simulink model "Male_female"  (R2017a)
settings: Solver=VariableStepAuto  StartTime=0.0  StopTime=10.0  RelTol=1e-3
libraries: dspvision x1
settings Model: Creator=harsh  LastModifiedBy=harsh

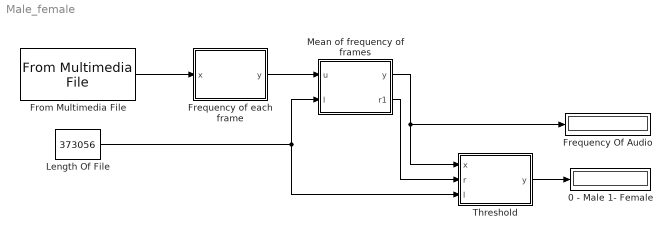
== system Male_female ==
  0 - Male 1- Female : Display
  Frequency Of Audio : Display
  Frequency of each frame : MATLAB Function  TreatAsAtomicUnit=on
  From Multimedia File : dspvision/From Multimedia File  inputFilename=E:\LNMIIT Study\Sem 5\Labs\DSP\Website\DSP Lab\Project (Male - Female Voice Recognition)\Project\samples\m2.wav  loop=on  numPlays=inf  outputStreams=Audio only  videoDataType=single  audioDataType=single  inheritSampleTime=on  userDefinedSampleTime=1/30  noAudioOutput=off  isIntensityVideo=off  fourcc=RGB  colorVideoFormat=Separate color signals  outputEOF=off  dataOrg=Column-major  audioFrameSize=3500  computeAudioFrameSize=off  outSamplingMode=Sample based
      settings: SourceProductBaseCode=VP
  "Length Of File " : Constant  Value=373056
  Mean of frequency of frames : MATLAB Function  TreatAsAtomicUnit=on
  Threshold : MATLAB Function  TreatAsAtomicUnit=on
  wires:
  From Multimedia File/1 -> Frequency of each frame/1(x)
  Frequency of each frame/1(y) -> Mean of frequency of frames/1(u)
  Mean of frequency of frames/1(y) -> Frequency Of Audio/1, Threshold/1(x)
  "Length Of File "/1 -> Threshold/3(l), Mean of frequency of frames/2(l)
  Threshold/1(y) -> 0 - Male 1- Female/1
  Mean of frequency of frames/2(r1) -> Threshold/2(r)

== matlab function Male_female/Threshold ==
  data: x input; r input; y output; l input
function y = fcn(x,r,l)
y=5;
if r>l/3500
    if x>160
        y=1;
    else
        y=0;
    end
end
end

== matlab function Male_female/Frequency of each frame ==
  data: x input; y output
function y = fcn(x)
Fs=44100;
coder.extrinsic('butter');
coder.extrinsic('filter');
[b0,a0]=butter(2,325/(Fs/2));
xin = abs(x);
xin=filter(b0,a0,xin);
xin = xin-mean(xin);
x2=zeros(length(xin),1);
x2(1:length(x)-1)=xin(2:length(x));
zc=length(find((xin>0 & x2<0) | (xin<0 & x2>0)));
y = 0.5*Fs*zc/length(x);

== matlab function Male_female/Mean of frequency of frames ==
  data: u input; y output; l input; r1 output
function [y,r1] = fcn(u,l)
persistent i
persistent r
if isempty(i)
        i = 0;
end
if isempty(r)
        r = 0;
end
j=l/3500;
i= (u/j)+i;
r=r+1;
r1=r;
y = i;
